simulink model "test_mdl1"  (R2023a)
settings: Solver=VariableStepAuto  StartTime=0.0  StopTime=10.0  RelTol=1e-3
(part 1 of 8)
settings Model: Creator=smqwzy  LastModifiedBy=smqwzy

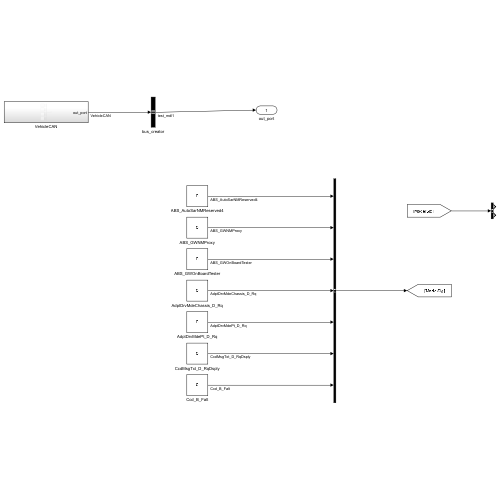
[thumbnail: Simulink's stored preview of the top-level diagram]
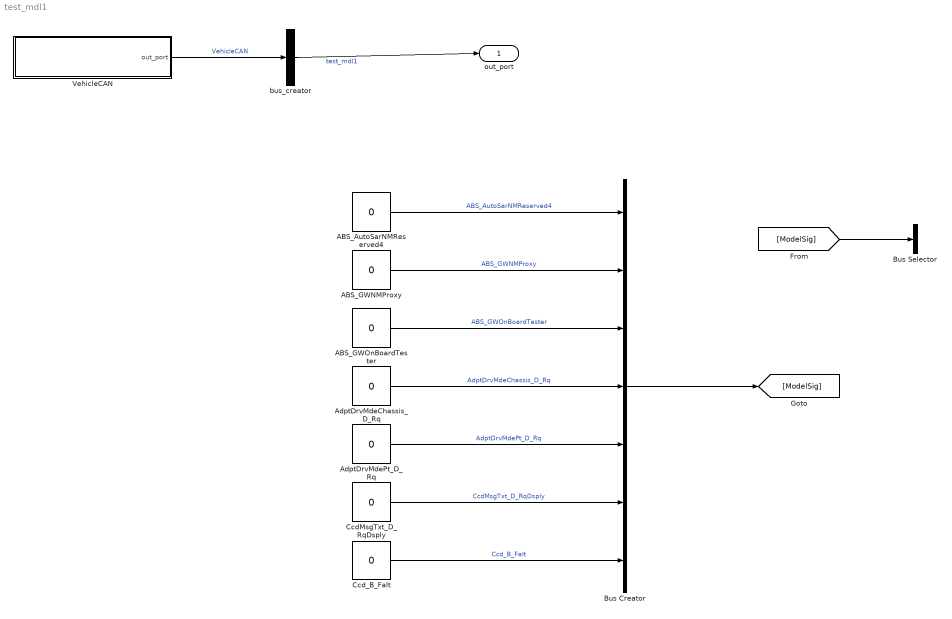
== system test_mdl1 ==
  ABS_AutoSarNMReserved4 : Constant  Value=0
  ABS_GWNMProxy : Constant  Value=0
  ABS_GWOnBoardTester : Constant  Value=0
  AdptDrvMdeChassis_D_Rq : Constant  Value=0
  AdptDrvMdePt_D_Rq : Constant  Value=0
  Bus Creator : BusCreator  Inputs=7
  Bus Selector : BusSelector  OutputSignals=signal1,signal2
  CcdMsgTxt_D_RqDsply : Constant  Value=0
  Ccd_B_Falt : Constant  Value=0
  VehicleCAN : Subsystem
  bus_creator : BusCreator  Inputs=1
  out_port : Outport
  wires:
  bus_creator/1 -> out_port/1  "test_mdl1"
  VehicleCAN/1(out_port) -> bus_creator/1  "VehicleCAN"
  Bus Creator/1 -> [ModelSig]
  [ModelSig] -> Bus Selector/1
  ABS_GWNMProxy/1 -> Bus Creator/2  "ABS_GWNMProxy"
  ABS_GWOnBoardTester/1 -> Bus Creator/3  "ABS_GWOnBoardTester"
  AdptDrvMdeChassis_D_Rq/1 -> Bus Creator/4  "AdptDrvMdeChassis_D_Rq"
  AdptDrvMdePt_D_Rq/1 -> Bus Creator/5  "AdptDrvMdePt_D_Rq"
  CcdMsgTxt_D_RqDsply/1 -> Bus Creator/6  "CcdMsgTxt_D_RqDsply"
  Ccd_B_Falt/1 -> Bus Creator/7  "Ccd_B_Falt"
  ABS_AutoSarNMReserved4/1 -> Bus Creator/1  "ABS_AutoSarNMReserved4"

== system test_mdl1/VehicleCAN ==
  ABS_ESC : Subsystem
  CMR_DSMC : Subsystem
  ECM_Diesel : Subsystem
  GWM : Subsystem
  IPMA_ADAS : Subsystem
  PCM : Subsystem
  PCM_HEV : Subsystem
  PSCM : Subsystem
  SOBDMC_HPCM_FD1 : Subsystem
  TCCM : Subsystem
  TCM_DSL : Subsystem
  TSTR : Subsystem
  VDM : Subsystem
  bus_creator : BusCreator  Inputs=13
  out_port : Outport
  wires:
  bus_creator/1 -> out_port/1  "test_mdl1"
  ABS_ESC/1(out_port) -> bus_creator/1  "ABS_ESC"
  CMR_DSMC/1(out_port) -> bus_creator/2  "CMR_DSMC"
  ECM_Diesel/1(out_port) -> bus_creator/3  "ECM_Diesel"
  GWM/1(out_port) -> bus_creator/4  "GWM"
  IPMA_ADAS/1(out_port) -> bus_creator/5  "IPMA_ADAS"
  PCM/1(out_port) -> bus_creator/6  "PCM"
  PCM_HEV/1(out_port) -> bus_creator/7  "PCM_HEV"
  PSCM/1(out_port) -> bus_creator/8  "PSCM"
  SOBDMC_HPCM_FD1/1(out_port) -> bus_creator/9  "SOBDMC_HPCM_FD1"
  TCCM/1(out_port) -> bus_creator/10  "TCCM"
  TCM_DSL/1(out_port) -> bus_creator/11  "TCM_DSL"
  TSTR/1(out_port) -> bus_creator/12  "TSTR"
  VDM/1(out_port) -> bus_creator/13  "VDM"

== system test_mdl1/VehicleCAN/ABS_ESC ==
  ABS_AutoSar_NetworkMgt : Subsystem
  ABS_BrkBst_Data : Subsystem
  ABS_Rapid_Data_Response_1 : Subsystem
  ABS_Rapid_Data_Response_2 : Subsystem
  ActiveFronSteering_Req : Subsystem
  BrakeSnData_3 : Subsystem
  BrakeSnData_4 : Subsystem
  BrakeSnData_5 : Subsystem
  BrakeSnData_6 : Subsystem
  BrakeSysFeatures : Subsystem
  BrakeSysFeatures_2 : Subsystem
  BrakeSysFeatures_3 : Subsystem
  DesiredTorqBrk : Subsystem
  DesiredTorqBrk_2 : Subsystem
  Global_PATS_SubTarget : Subsystem
  OTAPhysABStoGWM_ECG : Subsystem
  PARSEDPhysABStoGWM_ECG : Subsystem
  PARSEDPushABStoGWM_ECG : Subsystem
  SelectDriveModeData : Subsystem
  SelectDriveModeData2 : Subsystem
  TesterPhysicalResABS : Subsystem
  TrailerBrakeData : Subsystem
  WheelData : Subsystem
  WheelSpeed : Subsystem
  bus_creator : BusCreator  Inputs=24
  out_port : Outport
  wires:
  bus_creator/1 -> out_port/1  "test_mdl1"
  ABS_AutoSar_NetworkMgt/1(out_port) -> bus_creator/1  "ABS_AutoSar_NetworkMgt"
  ABS_BrkBst_Data/1(out_port) -> bus_creator/2  "ABS_BrkBst_Data"
  ABS_Rapid_Data_Response_1/1(out_port) -> bus_creator/3  "ABS_Rapid_Data_Response_1"
  ABS_Rapid_Data_Response_2/1(out_port) -> bus_creator/4  "ABS_Rapid_Data_Response_2"
  ActiveFronSteering_Req/1(out_port) -> bus_creator/5  "ActiveFronSteering_Req"
  BrakeSnData_3/1(out_port) -> bus_creator/6  "BrakeSnData_3"
  BrakeSnData_4/1(out_port) -> bus_creator/7  "BrakeSnData_4"
  BrakeSnData_5/1(out_port) -> bus_creator/8  "BrakeSnData_5"
  BrakeSnData_6/1(out_port) -> bus_creator/9  "BrakeSnData_6"
  BrakeSysFeatures/1(out_port) -> bus_creator/10  "BrakeSysFeatures"
  BrakeSysFeatures_2/1(out_port) -> bus_creator/11  "BrakeSysFeatures_2"
  BrakeSysFeatures_3/1(out_port) -> bus_creator/12  "BrakeSysFeatures_3"
  DesiredTorqBrk/1(out_port) -> bus_creator/13  "DesiredTorqBrk"
  DesiredTorqBrk_2/1(out_port) -> bus_creator/14  "DesiredTorqBrk_2"
  Global_PATS_SubTarget/1(out_port) -> bus_creator/15  "Global_PATS_SubTarget"
  OTAPhysABStoGWM_ECG/1(out_port) -> bus_creator/16  "OTAPhysABStoGWM_ECG"
  PARSEDPhysABStoGWM_ECG/1(out_port) -> bus_creator/17  "PARSEDPhysABStoGWM_ECG"
  PARSEDPushABStoGWM_ECG/1(out_port) -> bus_creator/18  "PARSEDPushABStoGWM_ECG"
  SelectDriveModeData/1(out_port) -> bus_creator/19  "SelectDriveModeData"
  SelectDriveModeData2/1(out_port) -> bus_creator/20  "SelectDriveModeData2"
  TesterPhysicalResABS/1(out_port) -> bus_creator/21  "TesterPhysicalResABS"
  TrailerBrakeData/1(out_port) -> bus_creator/22  "TrailerBrakeData"
  WheelData/1(out_port) -> bus_creator/23  "WheelData"
  WheelSpeed/1(out_port) -> bus_creator/24  "WheelSpeed"

== system test_mdl1/VehicleCAN/CMR_DSMC ==
  CMR_DSMC_AutoSar_NetwrkMgt : Subsystem
  DrvStatMonData : Subsystem
  TesterPhysicalResCMR_DSMC : Subsystem
  bus_creator : BusCreator  Inputs=3
  out_port : Outport
  wires:
  bus_creator/1 -> out_port/1  "test_mdl1"
  CMR_DSMC_AutoSar_NetwrkMgt/1(out_port) -> bus_creator/1  "CMR_DSMC_AutoSar_NetwrkMgt"
  DrvStatMonData/1(out_port) -> bus_creator/2  "DrvStatMonData"
  TesterPhysicalResCMR_DSMC/1(out_port) -> bus_creator/3  "TesterPhysicalResCMR_DSMC"

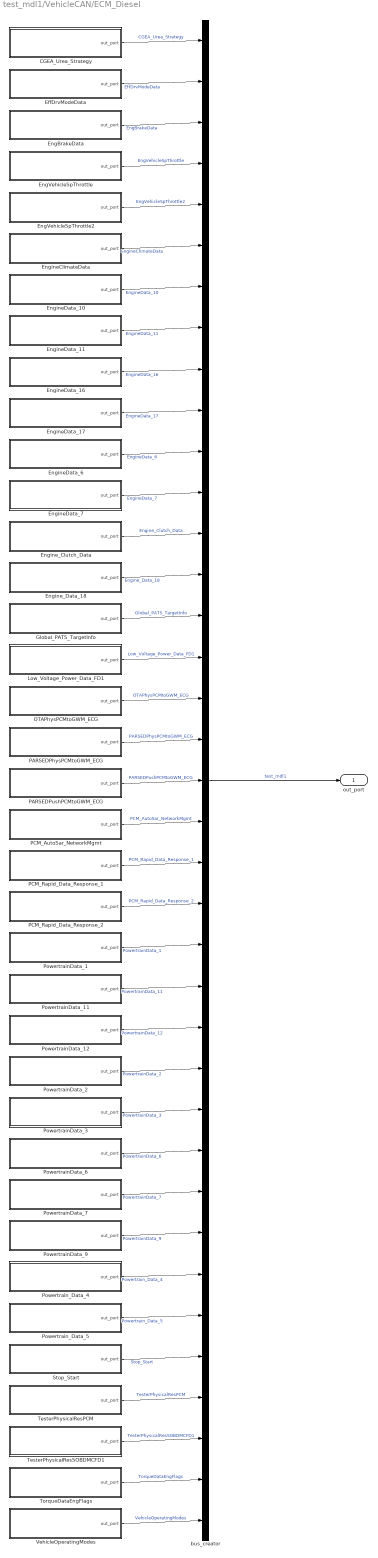
== system test_mdl1/VehicleCAN/ECM_Diesel ==
  CGEA_Urea_Strategy : Subsystem
  EffDrvModeData : Subsystem
  EngBrakeData : Subsystem
  EngVehicleSpThrottle : Subsystem
  EngVehicleSpThrottle2 : Subsystem
  EngineClimateData : Subsystem
  EngineData_10 : Subsystem
  EngineData_11 : Subsystem
  EngineData_16 : Subsystem
  EngineData_17 : Subsystem
  EngineData_6 : Subsystem
  EngineData_7 : Subsystem
  Engine_Clutch_Data : Subsystem
  Engine_Data_18 : Subsystem
  Global_PATS_TargetInfo : Subsystem
  Low_Voltage_Power_Data_FD1 : Subsystem
  OTAPhysPCMtoGWM_ECG : Subsystem
  PARSEDPhysPCMtoGWM_ECG : Subsystem
  PARSEDPushPCMtoGWM_ECG : Subsystem
  PCM_AutoSar_NetworkMgmt : Subsystem
  PCM_Rapid_Data_Response_1 : Subsystem
  PCM_Rapid_Data_Response_2 : Subsystem
  PowertrainData_1 : Subsystem
  PowertrainData_11 : Subsystem
  PowertrainData_12 : Subsystem
  PowertrainData_2 : Subsystem
  PowertrainData_3 : Subsystem
  PowertrainData_6 : Subsystem
  PowertrainData_7 : Subsystem
  PowertrainData_9 : Subsystem
  Powertrain_Data_4 : Subsystem
  Powertrain_Data_5 : Subsystem
  Stop_Start : Subsystem
  TesterPhysicalResPCM : Subsystem
  TesterPhysicalResSOBDMCFD1 : Subsystem
  TorqueDataEngFlags : Subsystem
  VehicleOperatingModes : Subsystem
  bus_creator : BusCreator  Inputs=37
  out_port : Outport
  wires:
  bus_creator/1 -> out_port/1  "test_mdl1"
  CGEA_Urea_Strategy/1(out_port) -> bus_creator/1  "CGEA_Urea_Strategy"
  EffDrvModeData/1(out_port) -> bus_creator/2  "EffDrvModeData"
  EngBrakeData/1(out_port) -> bus_creator/3  "EngBrakeData"
  EngVehicleSpThrottle/1(out_port) -> bus_creator/4  "EngVehicleSpThrottle"
  EngVehicleSpThrottle2/1(out_port) -> bus_creator/5  "EngVehicleSpThrottle2"
  EngineClimateData/1(out_port) -> bus_creator/6  "EngineClimateData"
  EngineData_10/1(out_port) -> bus_creator/7  "EngineData_10"
  EngineData_11/1(out_port) -> bus_creator/8  "EngineData_11"
  EngineData_16/1(out_port) -> bus_creator/9  "EngineData_16"
  EngineData_17/1(out_port) -> bus_creator/10  "EngineData_17"
  EngineData_6/1(out_port) -> bus_creator/11  "EngineData_6"
  EngineData_7/1(out_port) -> bus_creator/12  "EngineData_7"
  Engine_Clutch_Data/1(out_port) -> bus_creator/13  "Engine_Clutch_Data"
  Engine_Data_18/1(out_port) -> bus_creator/14  "Engine_Data_18"
  Global_PATS_TargetInfo/1(out_port) -> bus_creator/15  "Global_PATS_TargetInfo"
  Low_Voltage_Power_Data_FD1/1(out_port) -> bus_creator/16  "Low_Voltage_Power_Data_FD1"
  OTAPhysPCMtoGWM_ECG/1(out_port) -> bus_creator/17  "OTAPhysPCMtoGWM_ECG"
  PARSEDPhysPCMtoGWM_ECG/1(out_port) -> bus_creator/18  "PARSEDPhysPCMtoGWM_ECG"
  PARSEDPushPCMtoGWM_ECG/1(out_port) -> bus_creator/19  "PARSEDPushPCMtoGWM_ECG"
  PCM_AutoSar_NetworkMgmt/1(out_port) -> bus_creator/20  "PCM_AutoSar_NetworkMgmt"
  PCM_Rapid_Data_Response_1/1(out_port) -> bus_creator/21  "PCM_Rapid_Data_Response_1"
  PCM_Rapid_Data_Response_2/1(out_port) -> bus_creator/22  "PCM_Rapid_Data_Response_2"
  PowertrainData_1/1(out_port) -> bus_creator/23  "PowertrainData_1"
  PowertrainData_11/1(out_port) -> bus_creator/24  "PowertrainData_11"
  PowertrainData_12/1(out_port) -> bus_creator/25  "PowertrainData_12"
  PowertrainData_2/1(out_port) -> bus_creator/26  "PowertrainData_2"
  PowertrainData_3/1(out_port) -> bus_creator/27  "PowertrainData_3"
  PowertrainData_6/1(out_port) -> bus_creator/28  "PowertrainData_6"
  PowertrainData_7/1(out_port) -> bus_creator/29  "PowertrainData_7"
  PowertrainData_9/1(out_port) -> bus_creator/30  "PowertrainData_9"
  Powertrain_Data_4/1(out_port) -> bus_creator/31  "Powertrain_Data_4"
  Powertrain_Data_5/1(out_port) -> bus_creator/32  "Powertrain_Data_5"
  Stop_Start/1(out_port) -> bus_creator/33  "Stop_Start"
  TesterPhysicalResPCM/1(out_port) -> bus_creator/34  "TesterPhysicalResPCM"
  TesterPhysicalResSOBDMCFD1/1(out_port) -> bus_creator/35  "TesterPhysicalResSOBDMCFD1"
  TorqueDataEngFlags/1(out_port) -> bus_creator/36  "TorqueDataEngFlags"
  VehicleOperatingModes/1(out_port) -> bus_creator/37  "VehicleOperatingModes"

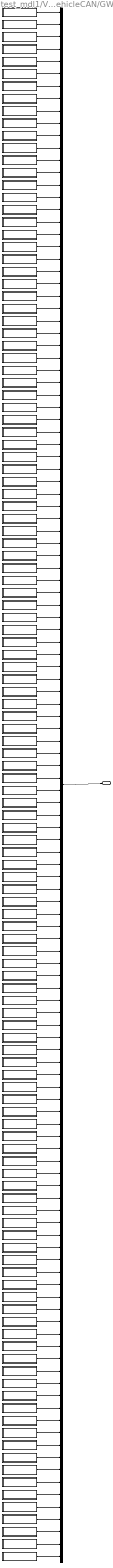
== system test_mdl1/VehicleCAN/GWM ==
  %sonality_APIM_Data_FD1 : Subsystem
  %sonality_BCM2_Data_FD1 : Subsystem
  %sonality_Data_FD1 : Subsystem
  AC_Compressor_Data_FD1 : Subsystem
  APIMGPS_Data_Nav_1_FD1 : Subsystem
  APIMGPS_Data_Nav_2_FD1 : Subsystem
  APIMGPS_Data_Nav_3_FD1 : Subsystem
  APIM_Data_FD1 : Subsystem
  APIM_Request_Signals_1_FD1 : Subsystem
  APIM_Request_Signals_5_FD1 : Subsystem
  APIM_Request_Signals_FD1 : Subsystem
  APIM_Send_Signals1_FD1 : Subsystem
  APIM_Send_Signals_2_FD1 : Subsystem
  Accel_Data_FD1 : Subsystem
  ActiveFrontStrg_Stat2_FD1 : Subsystem
  ActiveFrontStrg_Stat_FD1 : Subsystem
  Adaptive_Headlamp_Stat : Subsystem
  AllTerrainControlData_FD1 : Subsystem
  All_Terrain_Data_FD1 : Subsystem
  BCMC_Data_FD1 : Subsystem
  BCM_Lamp_Stat_FD1 : Subsystem
  BattRgenLo_1_FD1 : Subsystem
  BattRgenLo_2_FD1 : Subsystem
  BattRgenLo_3_FD1 : Subsystem
  BattRgenLo_4_FD1 : Subsystem
  Battery_Mgmt_24V_FD1 : Subsystem
  Battery_Mgmt_2_FD1 : Subsystem
  Battery_Mgmt_3_FD1 : Subsystem
  Battery_Mgmt_4_FD1 : Subsystem
  Battery_Traction_1_FD1 : Subsystem
  Battery_Traction_3_FD1 : Subsystem
  Battery_Traction_4_FD1 : Subsystem
  Battery_Traction_5_FD1 : Subsystem
  Battery_Traction_6_FD1 : Subsystem
  BodyInfo_3_FD1 : Subsystem
  Body_Info_10_FD1 : Subsystem
  Body_Info_4_FD1 : Subsystem
  Body_Info_6_FD1 : Subsystem
  Body_Info_8_FD1 : Subsystem
  Body_Info_9_FD1 : Subsystem
  Climate_Cntrl_Data_2_FD1 : Subsystem
  Climate_Control_Data_FD1 : Subsystem
  Cluster_HEV_Data8_FD1 : Subsystem
  Cluster_Info1_FD1 : Subsystem
  Cluster_Info_3_FD1 : Subsystem
  Cluster_Lighting_Rq_FD1 : Subsystem
  Compressor_Req_FD1 : Subsystem
  CruiseCtrl_Strg_Data_FD1 : Subsystem
  DCACA_Data1_FD1 : Subsystem
  DCACA_Data2_FD1 : Subsystem
  DCACA_Data3_FD1 : Subsystem
  DTE_ECGtoHPCM : Subsystem
  Driver_Dr_Stat_FD1 : Subsystem
  Dsp_Request_Signals11_FD1 : Subsystem
  ECG_Data2_FD1 : Subsystem
  ECG_Data3_FD1 : Subsystem
  ECG_Data4_FD1 : Subsystem
  ECG_Data_FD1 : Subsystem
  ElecHorizon_Data1_FD1 : Subsystem
  ElecHorizon_Data2_FD1 : Subsystem
  FourByFourSwitchData_FD1 : Subsystem
  GGCC_Config_Mgmt_ID_1_FD1 : Subsystem
  GWM_AutoSar_NetMgmt_FD1 : Subsystem
  Gear_Shift_by_Wire_2_FD1 : Subsystem
  Gear_Shift_by_Wire_FD1 : Subsystem
  GlobalClock_Data_FD1 : Subsystem
  Global_PATS_Cntrl_Info_FD1 : Subsystem
  Global_PATS_Ctrl_Info2_FD1 : Subsystem
  HeadUpDisplayReq_FD1 : Subsystem
  IPC_Infotainment_FD1 : Subsystem
  IPC_Send_Signals_2_FD1 : Subsystem
  LocationServices_3_FD1 : Subsystem
  LocationServices_Data1_FD1 : Subsystem
  Locking_Systems_2_FD1 : Subsystem
  MasterReset_HS3_ECGDat_FD1 : Subsystem
  Mc_Send_Signals_2_FD1 : Subsystem
  OTAFuncGWM_ECG_FD1 : Subsystem
  OTAPhysGWM_ECGtoABS : Subsystem
  OTAPhysGWM_ECGtoCCM : Subsystem
  OTAPhysGWM_ECGtoIPMA : Subsystem
  OTAPhysGWM_ECGtoPCM : Subsystem
  OTAPhysGWM_ECGtoSOBDMC_FD1 : Subsystem
  OTAPhysGWM_ECGtoSODCMC : Subsystem
  OTAPhysGWM_ECGtoSODCMD : Subsystem
  OTAPhysGWM_ECGtoSODL : Subsystem
  OTAPhysGWM_ECGtoSODR : Subsystem
  OffBrdChrg_Signals : Subsystem
  OffBrdChrg_Signals2 : Subsystem
  PARSEDFuncGWM_ECG_FD1 : Subsystem
  PARSEDPhysGWM_ECGtoABS : Subsystem
  PARSEDPhysGWM_ECGtoCCM : Subsystem
  PARSEDPhysGWM_ECGtoIPMA : Subsystem
  PARSEDPhysGWM_ECGtoPCM : Subsystem
  PARSEDPhysGWM_ECGtoSODCMC : Subsystem
  PARSEDPhysGWM_ECGtoSODCMD : Subsystem
  PARSEDPhysGWM_ECGtoSODL : Subsystem
  PARSEDPhysGWM_ECGtoSODR : Subsystem
  PARSEDPhysGWMtoSOBDMC_FD1 : Subsystem
  PARSEDPushFcGWM_ECGtoABS : Subsystem
  PARSEDPushFcGWM_ECGtoPCM : Subsystem
  PHEV_Battery_Data1_FD1 : Subsystem
  ParkAid_Aud_Warn_CmdM_FD1 : Subsystem
  Pass_Dr_Stat_FD1 : Subsystem
  PowerDistData_2_FD1 : Subsystem
  PowerDist_Data1_FD1 : Subsystem
  Power_Liftgate_Stat_FD1 : Subsystem
  RCMSerialNumber_FD1 : Subsystem
  RCMStatusMessage2_FD1 : Subsystem
  SmartChargingData_ECG_1 : Subsystem
  SmartChargingData_ECG_2 : Subsystem
  SmartChargingData_ECG_3 : Subsystem
  Steering_Data_FD1 : Subsystem
  Steering_Wheel_Data2_FD1 : Subsystem
  TCU_Send_Signals_FD1 : Subsystem
  TesterPhysicalReqVDM_FD1 : Subsystem
  TesterPhysicalResGWM_FD1 : Subsystem
  Tire_Pressure_Data_FD1 : Subsystem
  TrailerAid_Data3_FD1 : Subsystem
  TrailerAid_Data_FD1 : Subsystem
  TrailerAid_Stat1_FD1 : Subsystem
  TrailerAid_Stat2_FD1 : Subsystem
  TrailerBrakeInfo_FD1 : Subsystem
  TrailerInfo_2_FD1 : Subsystem
  TrailerInfo_FD1 : Subsystem
  Voltage_Power_Data2_FD1 : Subsystem
  Yaw_Data_FD1 : Subsystem
  bus_creator : BusCreator  Inputs=126
  out_port : Outport
  wires:
  bus_creator/1 -> out_port/1  "test_mdl1"
  AC_Compressor_Data_FD1/1(out_port) -> bus_creator/1  "AC_Compressor_Data_FD1"
  APIMGPS_Data_Nav_1_FD1/1(out_port) -> bus_creator/2  "APIMGPS_Data_Nav_1_FD1"
  APIMGPS_Data_Nav_2_FD1/1(out_port) -> bus_creator/3  "APIMGPS_Data_Nav_2_FD1"
  APIMGPS_Data_Nav_3_FD1/1(out_port) -> bus_creator/4  "APIMGPS_Data_Nav_3_FD1"
  APIM_Data_FD1/1(out_port) -> bus_creator/5  "APIM_Data_FD1"
  APIM_Request_Signals_1_FD1/1(out_port) -> bus_creator/6  "APIM_Request_Signals_1_FD1"
  APIM_Request_Signals_5_FD1/1(out_port) -> bus_creator/7  "APIM_Request_Signals_5_FD1"
  APIM_Request_Signals_FD1/1(out_port) -> bus_creator/8  "APIM_Request_Signals_FD1"
  APIM_Send_Signals1_FD1/1(out_port) -> bus_creator/9  "APIM_Send_Signals1_FD1"
  APIM_Send_Signals_2_FD1/1(out_port) -> bus_creator/10  "APIM_Send_Signals_2_FD1"
  Accel_Data_FD1/1(out_port) -> bus_creator/11  "Accel_Data_FD1"
  ActiveFrontStrg_Stat2_FD1/1(out_port) -> bus_creator/12  "ActiveFrontStrg_Stat2_FD1"
  ActiveFrontStrg_Stat_FD1/1(out_port) -> bus_creator/13  "ActiveFrontStrg_Stat_FD1"
  Adaptive_Headlamp_Stat/1(out_port) -> bus_creator/14  "Adaptive_Headlamp_Stat"
  AllTerrainControlData_FD1/1(out_port) -> bus_creator/15  "AllTerrainControlData_FD1"
  All_Terrain_Data_FD1/1(out_port) -> bus_creator/16  "All_Terrain_Data_FD1"
  BCMC_Data_FD1/1(out_port) -> bus_creator/17  "BCMC_Data_FD1"
  BCM_Lamp_Stat_FD1/1(out_port) -> bus_creator/18  "BCM_Lamp_Stat_FD1"
  BattRgenLo_1_FD1/1(out_port) -> bus_creator/19  "BattRgenLo_1_FD1"
  BattRgenLo_2_FD1/1(out_port) -> bus_creator/20  "BattRgenLo_2_FD1"
  BattRgenLo_3_FD1/1(out_port) -> bus_creator/21  "BattRgenLo_3_FD1"
  BattRgenLo_4_FD1/1(out_port) -> bus_creator/22  "BattRgenLo_4_FD1"
  Battery_Mgmt_24V_FD1/1(out_port) -> bus_creator/23  "Battery_Mgmt_24V_FD1"
  Battery_Mgmt_2_FD1/1(out_port) -> bus_creator/24  "Battery_Mgmt_2_FD1"
  Battery_Mgmt_3_FD1/1(out_port) -> bus_creator/25  "Battery_Mgmt_3_FD1"
  Battery_Mgmt_4_FD1/1(out_port) -> bus_creator/26  "Battery_Mgmt_4_FD1"
  Battery_Traction_1_FD1/1(out_port) -> bus_creator/27  "Battery_Traction_1_FD1"
  Battery_Traction_3_FD1/1(out_port) -> bus_creator/28  "Battery_Traction_3_FD1"
  Battery_Traction_4_FD1/1(out_port) -> bus_creator/29  "Battery_Traction_4_FD1"
  Battery_Traction_5_FD1/1(out_port) -> bus_creator/30  "Battery_Traction_5_FD1"
  Battery_Traction_6_FD1/1(out_port) -> bus_creator/31  "Battery_Traction_6_FD1"
  BodyInfo_3_FD1/1(out_port) -> bus_creator/32  "BodyInfo_3_FD1"
  Body_Info_10_FD1/1(out_port) -> bus_creator/33  "Body_Info_10_FD1"
  Body_Info_4_FD1/1(out_port) -> bus_creator/34  "Body_Info_4_FD1"
  Body_Info_6_FD1/1(out_port) -> bus_creator/35  "Body_Info_6_FD1"
  Body_Info_8_FD1/1(out_port) -> bus_creator/36  "Body_Info_8_FD1"
  Body_Info_9_FD1/1(out_port) -> bus_creator/37  "Body_Info_9_FD1"
  Climate_Cntrl_Data_2_FD1/1(out_port) -> bus_creator/38  "Climate_Cntrl_Data_2_FD1"
  Climate_Control_Data_FD1/1(out_port) -> bus_creator/39  "Climate_Control_Data_FD1"
  Cluster_HEV_Data8_FD1/1(out_port) -> bus_creator/40  "Cluster_HEV_Data8_FD1"
  Cluster_Info1_FD1/1(out_port) -> bus_creator/41  "Cluster_Info1_FD1"
  Cluster_Info_3_FD1/1(out_port) -> bus_creator/42  "Cluster_Info_3_FD1"
  Cluster_Lighting_Rq_FD1/1(out_port) -> bus_creator/43  "Cluster_Lighting_Rq_FD1"
  Compressor_Req_FD1/1(out_port) -> bus_creator/44  "Compressor_Req_FD1"
  CruiseCtrl_Strg_Data_FD1/1(out_port) -> bus_creator/45  "CruiseCtrl_Strg_Data_FD1"
  DCACA_Data1_FD1/1(out_port) -> bus_creator/46  "DCACA_Data1_FD1"
  DCACA_Data2_FD1/1(out_port) -> bus_creator/47  "DCACA_Data2_FD1"
  DCACA_Data3_FD1/1(out_port) -> bus_creator/48  "DCACA_Data3_FD1"
  DTE_ECGtoHPCM/1(out_port) -> bus_creator/49  "DTE_ECGtoHPCM"
  Driver_Dr_Stat_FD1/1(out_port) -> bus_creator/50  "Driver_Dr_Stat_FD1"
  Dsp_Request_Signals11_FD1/1(out_port) -> bus_creator/51  "Dsp_Request_Signals11_FD1"
  ECG_Data2_FD1/1(out_port) -> bus_creator/52  "ECG_Data2_FD1"
  ECG_Data3_FD1/1(out_port) -> bus_creator/53  "ECG_Data3_FD1"
  ECG_Data4_FD1/1(out_port) -> bus_creator/54  "ECG_Data4_FD1"
  ECG_Data_FD1/1(out_port) -> bus_creator/55  "ECG_Data_FD1"
  ElecHorizon_Data1_FD1/1(out_port) -> bus_creator/56  "ElecHorizon_Data1_FD1"
  ElecHorizon_Data2_FD1/1(out_port) -> bus_creator/57  "ElecHorizon_Data2_FD1"
  FourByFourSwitchData_FD1/1(out_port) -> bus_creator/58  "FourByFourSwitchData_FD1"
  GGCC_Config_Mgmt_ID_1_FD1/1(out_port) -> bus_creator/59  "GGCC_Config_Mgmt_ID_1_FD1"
  GWM_AutoSar_NetMgmt_FD1/1(out_port) -> bus_creator/60  "GWM_AutoSar_NetMgmt_FD1"
  Gear_Shift_by_Wire_2_FD1/1(out_port) -> bus_creator/61  "Gear_Shift_by_Wire_2_FD1"
  Gear_Shift_by_Wire_FD1/1(out_port) -> bus_creator/62  "Gear_Shift_by_Wire_FD1"
  GlobalClock_Data_FD1/1(out_port) -> bus_creator/63  "GlobalClock_Data_FD1"
  Global_PATS_Cntrl_Info_FD1/1(out_port) -> bus_creator/64  "Global_PATS_Cntrl_Info_FD1"
  Global_PATS_Ctrl_Info2_FD1/1(out_port) -> bus_creator/65  "Global_PATS_Ctrl_Info2_FD1"
  HeadUpDisplayReq_FD1/1(out_port) -> bus_creator/66  "HeadUpDisplayReq_FD1"
  IPC_Infotainment_FD1/1(out_port) -> bus_creator/67  "IPC_Infotainment_FD1"
  IPC_Send_Signals_2_FD1/1(out_port) -> bus_creator/68  "IPC_Send_Signals_2_FD1"
  LocationServices_3_FD1/1(out_port) -> bus_creator/69  "LocationServices_3_FD1"
  LocationServices_Data1_FD1/1(out_port) -> bus_creator/70  "LocationServices_Data1_FD1"
  Locking_Systems_2_FD1/1(out_port) -> bus_creator/71  "Locking_Systems_2_FD1"
  MasterReset_HS3_ECGDat_FD1/1(out_port) -> bus_creator/72  "MasterReset_HS3_ECGDat_FD1"
  Mc_Send_Signals_2_FD1/1(out_port) -> bus_creator/73  "Mc_Send_Signals_2_FD1"
  OTAFuncGWM_ECG_FD1/1(out_port) -> bus_creator/74  "OTAFuncGWM_ECG_FD1"
  OTAPhysGWM_ECGtoABS/1(out_port) -> bus_creator/75  "OTAPhysGWM_ECGtoABS"
  OTAPhysGWM_ECGtoCCM/1(out_port) -> bus_creator/76  "OTAPhysGWM_ECGtoCCM"
  OTAPhysGWM_ECGtoIPMA/1(out_port) -> bus_creator/77  "OTAPhysGWM_ECGtoIPMA"
  OTAPhysGWM_ECGtoPCM/1(out_port) -> bus_creator/78  "OTAPhysGWM_ECGtoPCM"
  OTAPhysGWM_ECGtoSOBDMC_FD1/1(out_port) -> bus_creator/79  "OTAPhysGWM_ECGtoSOBDMC_FD1"
  OTAPhysGWM_ECGtoSODCMC/1(out_port) -> bus_creator/80  "OTAPhysGWM_ECGtoSODCMC"
  OTAPhysGWM_ECGtoSODCMD/1(out_port) -> bus_creator/81  "OTAPhysGWM_ECGtoSODCMD"
  OTAPhysGWM_ECGtoSODL/1(out_port) -> bus_creator/82  "OTAPhysGWM_ECGtoSODL"
  OTAPhysGWM_ECGtoSODR/1(out_port) -> bus_creator/83  "OTAPhysGWM_ECGtoSODR"
  OffBrdChrg_Signals/1(out_port) -> bus_creator/84  "OffBrdChrg_Signals"
  OffBrdChrg_Signals2/1(out_port) -> bus_creator/85  "OffBrdChrg_Signals2"
  PARSEDFuncGWM_ECG_FD1/1(out_port) -> bus_creator/86  "PARSEDFuncGWM_ECG_FD1"
  PARSEDPhysGWM_ECGtoABS/1(out_port) -> bus_creator/87  "PARSEDPhysGWM_ECGtoABS"
  PARSEDPhysGWM_ECGtoCCM/1(out_port) -> bus_creator/88  "PARSEDPhysGWM_ECGtoCCM"
  PARSEDPhysGWM_ECGtoIPMA/1(out_port) -> bus_creator/89  "PARSEDPhysGWM_ECGtoIPMA"
  PARSEDPhysGWM_ECGtoPCM/1(out_port) -> bus_creator/90  "PARSEDPhysGWM_ECGtoPCM"
  PARSEDPhysGWM_ECGtoSODCMC/1(out_port) -> bus_creator/91  "PARSEDPhysGWM_ECGtoSODCMC"
  PARSEDPhysGWM_ECGtoSODCMD/1(out_port) -> bus_creator/92  "PARSEDPhysGWM_ECGtoSODCMD"
  PARSEDPhysGWM_ECGtoSODL/1(out_port) -> bus_creator/93  "PARSEDPhysGWM_ECGtoSODL"
  PARSEDPhysGWM_ECGtoSODR/1(out_port) -> bus_creator/94  "PARSEDPhysGWM_ECGtoSODR"
  PARSEDPhysGWMtoSOBDMC_FD1/1(out_port) -> bus_creator/95  "PARSEDPhysGWMtoSOBDMC_FD1"
  PARSEDPushFcGWM_ECGtoABS/1(out_port) -> bus_creator/96  "PARSEDPushFcGWM_ECGtoABS"
  PARSEDPushFcGWM_ECGtoPCM/1(out_port) -> bus_creator/97  "PARSEDPushFcGWM_ECGtoPCM"
  PHEV_Battery_Data1_FD1/1(out_port) -> bus_creator/98  "PHEV_Battery_Data1_FD1"
  ParkAid_Aud_Warn_CmdM_FD1/1(out_port) -> bus_creator/99  "ParkAid_Aud_Warn_CmdM_FD1"
  Pass_Dr_Stat_FD1/1(out_port) -> bus_creator/100  "Pass_Dr_Stat_FD1"
  %sonality_APIM_Data_FD1/1(out_port) -> bus_creator/101  "%sonality_APIM_Data_FD1"
  %sonality_BCM2_Data_FD1/1(out_port) -> bus_creator/102  "%sonality_BCM2_Data_FD1"
  %sonality_Data_FD1/1(out_port) -> bus_creator/103  "%sonality_Data_FD1"
  PowerDistData_2_FD1/1(out_port) -> bus_creator/104  "PowerDistData_2_FD1"
  PowerDist_Data1_FD1/1(out_port) -> bus_creator/105  "PowerDist_Data1_FD1"
  Power_Liftgate_Stat_FD1/1(out_port) -> bus_creator/106  "Power_Liftgate_Stat_FD1"
  RCMSerialNumber_FD1/1(out_port) -> bus_creator/107  "RCMSerialNumber_FD1"
  RCMStatusMessage2_FD1/1(out_port) -> bus_creator/108  "RCMStatusMessage2_FD1"
  SmartChargingData_ECG_1/1(out_port) -> bus_creator/109  "SmartChargingData_ECG_1"
  SmartChargingData_ECG_2/1(out_port) -> bus_creator/110  "SmartChargingData_ECG_2"
  SmartChargingData_ECG_3/1(out_port) -> bus_creator/111  "SmartChargingData_ECG_3"
  Steering_Data_FD1/1(out_port) -> bus_creator/112  "Steering_Data_FD1"
  Steering_Wheel_Data2_FD1/1(out_port) -> bus_creator/113  "Steering_Wheel_Data2_FD1"
  TCU_Send_Signals_FD1/1(out_port) -> bus_creator/114  "TCU_Send_Signals_FD1"
  TesterPhysicalReqVDM_FD1/1(out_port) -> bus_creator/115  "TesterPhysicalReqVDM_FD1"
  TesterPhysicalResGWM_FD1/1(out_port) -> bus_creator/116  "TesterPhysicalResGWM_FD1"
  Tire_Pressure_Data_FD1/1(out_port) -> bus_creator/117  "Tire_Pressure_Data_FD1"
  TrailerAid_Data3_FD1/1(out_port) -> bus_creator/118  "TrailerAid_Data3_FD1"
  TrailerAid_Data_FD1/1(out_port) -> bus_creator/119  "TrailerAid_Data_FD1"
  TrailerAid_Stat1_FD1/1(out_port) -> bus_creator/120  "TrailerAid_Stat1_FD1"
  TrailerAid_Stat2_FD1/1(out_port) -> bus_creator/121  "TrailerAid_Stat2_FD1"
  TrailerBrakeInfo_FD1/1(out_port) -> bus_creator/122  "TrailerBrakeInfo_FD1"
  TrailerInfo_2_FD1/1(out_port) -> bus_creator/123  "TrailerInfo_2_FD1"
  TrailerInfo_FD1/1(out_port) -> bus_creator/124  "TrailerInfo_FD1"
  Voltage_Power_Data2_FD1/1(out_port) -> bus_creator/125  "Voltage_Power_Data2_FD1"
  Yaw_Data_FD1/1(out_port) -> bus_creator/126  "Yaw_Data_FD1"

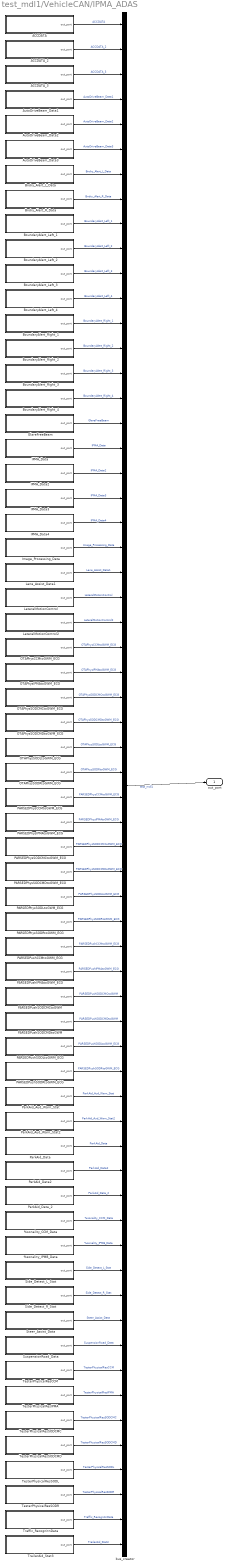
== system test_mdl1/VehicleCAN/IPMA_ADAS ==
  %sonality_CCM_Data : Subsystem
  %sonality_IPMB_Data : Subsystem
  ACCDATA : Subsystem
  ACCDATA_2 : Subsystem
  ACCDATA_3 : Subsystem
  AutoDriveBeam_Data1 : Subsystem
  AutoDriveBeam_Data2 : Subsystem
  AutoDriveBeam_Data3 : Subsystem
  Bndry_Alert_L_Data : Subsystem
  Bndry_Alert_R_Data : Subsystem
  BoundaryAlert_Left_1 : Subsystem
  BoundaryAlert_Left_2 : Subsystem
  BoundaryAlert_Left_3 : Subsystem
  BoundaryAlert_Left_4 : Subsystem
  BoundaryAlert_Right_1 : Subsystem
  BoundaryAlert_Right_2 : Subsystem
  BoundaryAlert_Right_3 : Subsystem
  BoundaryAlert_Right_4 : Subsystem
  GlareFreeBeam : Subsystem
  IPMA_Data : Subsystem
  IPMA_Data2 : Subsystem
  IPMA_Data3 : Subsystem
  IPMA_Data4 : Subsystem
  Image_Processing_Data : Subsystem
  Lane_Assist_Data1 : Subsystem
  LateralMotionControl : Subsystem
  LateralMotionControl2 : Subsystem
  OTAPhysCCMtoGWM_ECG : Subsystem
  OTAPhysIPMAtoGWM_ECG : Subsystem
  OTAPhysSODCMCtoGWM_ECG : Subsystem
  OTAPhysSODCMDtoGWM_ECG : Subsystem
  OTAPhysSODLtoGWM_ECG : Subsystem
  OTAPhysSODRtoGWM_ECG : Subsystem
  PARSEDPhysCCMtoGWM_ECG : Subsystem
  PARSEDPhysIPMAtoGWM_ECG : Subsystem
  PARSEDPhysSODCMCtoGWM_ECG : Subsystem
  PARSEDPhysSODCMDtoGWM_ECG : Subsystem
  PARSEDPhysSODLtoGWM_ECG : Subsystem
  PARSEDPhysSODRtoGWM_ECG : Subsystem
  PARSEDPushCCMtoGWM_ECG : Subsystem
  PARSEDPushIPMAtoGWM_ECG : Subsystem
  PARSEDPushSODCMCtoGWM : Subsystem
  PARSEDPushSODCMDtoGWM : Subsystem
  PARSEDPushSODLtoGWM_ECG : Subsystem
  PARSEDPushSODRtoGWM_ECG : Subsystem
  ParkAid_Aud_Warn_Stat : Subsystem
  ParkAid_Aud_Warn_Stat2 : Subsystem
  ParkAid_Data : Subsystem
  ParkAid_Data2 : Subsystem
  ParkAid_Data_2 : Subsystem
  Side_Detect_L_Stat : Subsystem
  Side_Detect_R_Stat : Subsystem
  Steer_Assist_Data : Subsystem
  SuspensionRoad_Data : Subsystem
  TesterPhysicalResCCM : Subsystem
  TesterPhysicalResIPMA : Subsystem
  TesterPhysicalResSODCMC : Subsystem
  TesterPhysicalResSODCMD : Subsystem
  TesterPhysicalResSODL : Subsystem
  TesterPhysicalResSODR : Subsystem
  Traffic_RecognitnData : Subsystem
  TrailerAid_Stat3 : Subsystem
  bus_creator : BusCreator  Inputs=62
  out_port : Outport
  wires:
  bus_creator/1 -> out_port/1  "test_mdl1"
  ACCDATA/1(out_port) -> bus_creator/1  "ACCDATA"
  ACCDATA_2/1(out_port) -> bus_creator/2  "ACCDATA_2"
  ACCDATA_3/1(out_port) -> bus_creator/3  "ACCDATA_3"
  AutoDriveBeam_Data1/1(out_port) -> bus_creator/4  "AutoDriveBeam_Data1"
  AutoDriveBeam_Data2/1(out_port) -> bus_creator/5  "AutoDriveBeam_Data2"
  AutoDriveBeam_Data3/1(out_port) -> bus_creator/6  "AutoDriveBeam_Data3"
  Bndry_Alert_L_Data/1(out_port) -> bus_creator/7  "Bndry_Alert_L_Data"
  Bndry_Alert_R_Data/1(out_port) -> bus_creator/8  "Bndry_Alert_R_Data"
  BoundaryAlert_Left_1/1(out_port) -> bus_creator/9  "BoundaryAlert_Left_1"
  BoundaryAlert_Left_2/1(out_port) -> bus_creator/10  "BoundaryAlert_Left_2"
  BoundaryAlert_Left_3/1(out_port) -> bus_creator/11  "BoundaryAlert_Left_3"
  BoundaryAlert_Left_4/1(out_port) -> bus_creator/12  "BoundaryAlert_Left_4"
  BoundaryAlert_Right_1/1(out_port) -> bus_creator/13  "BoundaryAlert_Right_1"
  BoundaryAlert_Right_2/1(out_port) -> bus_creator/14  "BoundaryAlert_Right_2"
  BoundaryAlert_Right_3/1(out_port) -> bus_creator/15  "BoundaryAlert_Right_3"
  BoundaryAlert_Right_4/1(out_port) -> bus_creator/16  "BoundaryAlert_Right_4"
  GlareFreeBeam/1(out_port) -> bus_creator/17  "GlareFreeBeam"
  IPMA_Data/1(out_port) -> bus_creator/18  "IPMA_Data"
  IPMA_Data2/1(out_port) -> bus_creator/19  "IPMA_Data2"
  IPMA_Data3/1(out_port) -> bus_creator/20  "IPMA_Data3"
  IPMA_Data4/1(out_port) -> bus_creator/21  "IPMA_Data4"
  Image_Processing_Data/1(out_port) -> bus_creator/22  "Image_Processing_Data"
  Lane_Assist_Data1/1(out_port) -> bus_creator/23  "Lane_Assist_Data1"
  LateralMotionControl/1(out_port) -> bus_creator/24  "LateralMotionControl"
  LateralMotionControl2/1(out_port) -> bus_creator/25  "LateralMotionControl2"
  OTAPhysCCMtoGWM_ECG/1(out_port) -> bus_creator/26  "OTAPhysCCMtoGWM_ECG"
  OTAPhysIPMAtoGWM_ECG/1(out_port) -> bus_creator/27  "OTAPhysIPMAtoGWM_ECG"
  OTAPhysSODCMCtoGWM_ECG/1(out_port) -> bus_creator/28  "OTAPhysSODCMCtoGWM_ECG"
  OTAPhysSODCMDtoGWM_ECG/1(out_port) -> bus_creator/29  "OTAPhysSODCMDtoGWM_ECG"
  OTAPhysSODLtoGWM_ECG/1(out_port) -> bus_creator/30  "OTAPhysSODLtoGWM_ECG"
  OTAPhysSODRtoGWM_ECG/1(out_port) -> bus_creator/31  "OTAPhysSODRtoGWM_ECG"
  PARSEDPhysCCMtoGWM_ECG/1(out_port) -> bus_creator/32  "PARSEDPhysCCMtoGWM_ECG"
  PARSEDPhysIPMAtoGWM_ECG/1(out_port) -> bus_creator/33  "PARSEDPhysIPMAtoGWM_ECG"
  PARSEDPhysSODCMCtoGWM_ECG/1(out_port) -> bus_creator/34  "PARSEDPhysSODCMCtoGWM_ECG"
  PARSEDPhysSODCMDtoGWM_ECG/1(out_port) -> bus_creator/35  "PARSEDPhysSODCMDtoGWM_ECG"
  PARSEDPhysSODLtoGWM_ECG/1(out_port) -> bus_creator/36  "PARSEDPhysSODLtoGWM_ECG"
  PARSEDPhysSODRtoGWM_ECG/1(out_port) -> bus_creator/37  "PARSEDPhysSODRtoGWM_ECG"
  PARSEDPushCCMtoGWM_ECG/1(out_port) -> bus_creator/38  "PARSEDPushCCMtoGWM_ECG"
  PARSEDPushIPMAtoGWM_ECG/1(out_port) -> bus_creator/39  "PARSEDPushIPMAtoGWM_ECG"
  PARSEDPushSODCMCtoGWM/1(out_port) -> bus_creator/40  "PARSEDPushSODCMCtoGWM"
  PARSEDPushSODCMDtoGWM/1(out_port) -> bus_creator/41  "PARSEDPushSODCMDtoGWM"
  PARSEDPushSODLtoGWM_ECG/1(out_port) -> bus_creator/42  "PARSEDPushSODLtoGWM_ECG"
  PARSEDPushSODRtoGWM_ECG/1(out_port) -> bus_creator/43  "PARSEDPushSODRtoGWM_ECG"
  ParkAid_Aud_Warn_Stat/1(out_port) -> bus_creator/44  "ParkAid_Aud_Warn_Stat"
  ParkAid_Aud_Warn_Stat2/1(out_port) -> bus_creator/45  "ParkAid_Aud_Warn_Stat2"
  ParkAid_Data/1(out_port) -> bus_creator/46  "ParkAid_Data"
  ParkAid_Data2/1(out_port) -> bus_creator/47  "ParkAid_Data2"
  ParkAid_Data_2/1(out_port) -> bus_creator/48  "ParkAid_Data_2"
  %sonality_CCM_Data/1(out_port) -> bus_creator/49  "%sonality_CCM_Data"
  %sonality_IPMB_Data/1(out_port) -> bus_creator/50  "%sonality_IPMB_Data"
  Side_Detect_L_Stat/1(out_port) -> bus_creator/51  "Side_Detect_L_Stat"
  Side_Detect_R_Stat/1(out_port) -> bus_creator/52  "Side_Detect_R_Stat"
  Steer_Assist_Data/1(out_port) -> bus_creator/53  "Steer_Assist_Data"
  SuspensionRoad_Data/1(out_port) -> bus_creator/54  "SuspensionRoad_Data"
  TesterPhysicalResCCM/1(out_port) -> bus_creator/55  "TesterPhysicalResCCM"
  TesterPhysicalResIPMA/1(out_port) -> bus_creator/56  "TesterPhysicalResIPMA"
  TesterPhysicalResSODCMC/1(out_port) -> bus_creator/57  "TesterPhysicalResSODCMC"
  TesterPhysicalResSODCMD/1(out_port) -> bus_creator/58  "TesterPhysicalResSODCMD"
  TesterPhysicalResSODL/1(out_port) -> bus_creator/59  "TesterPhysicalResSODL"
  TesterPhysicalResSODR/1(out_port) -> bus_creator/60  "TesterPhysicalResSODR"
  Traffic_RecognitnData/1(out_port) -> bus_creator/61  "Traffic_RecognitnData"
  TrailerAid_Stat3/1(out_port) -> bus_creator/62  "TrailerAid_Stat3"

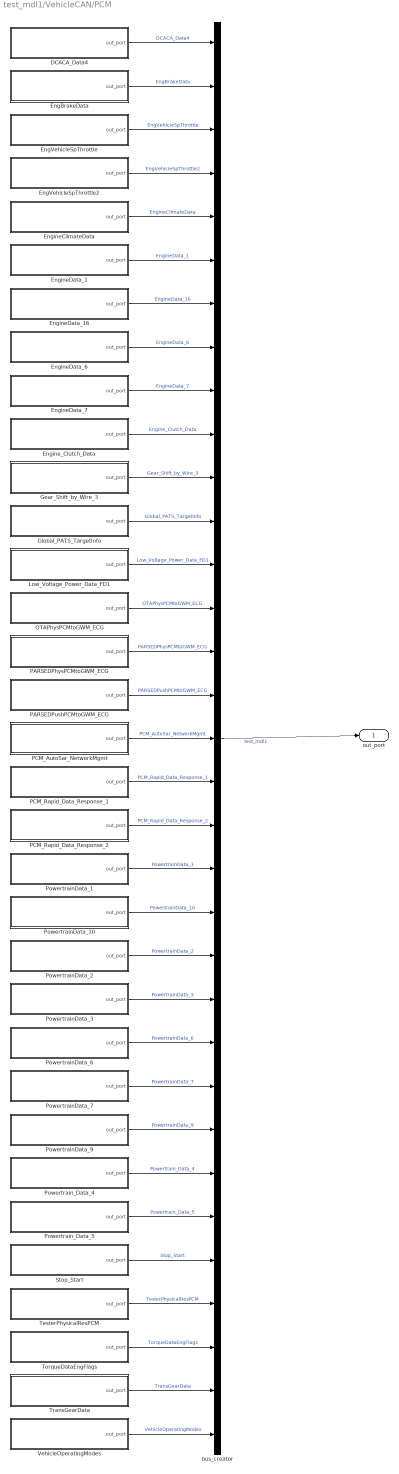
== system test_mdl1/VehicleCAN/PCM ==
  DCACA_Data4 : Subsystem
  EngBrakeData : Subsystem
  EngVehicleSpThrottle : Subsystem
  EngVehicleSpThrottle2 : Subsystem
  EngineClimateData : Subsystem
  EngineData_1 : Subsystem
  EngineData_16 : Subsystem
  EngineData_6 : Subsystem
  EngineData_7 : Subsystem
  Engine_Clutch_Data : Subsystem
  Gear_Shift_by_Wire_3 : Subsystem
  Global_PATS_TargetInfo : Subsystem
  Low_Voltage_Power_Data_FD1 : Subsystem
  OTAPhysPCMtoGWM_ECG : Subsystem
  PARSEDPhysPCMtoGWM_ECG : Subsystem
  PARSEDPushPCMtoGWM_ECG : Subsystem
  PCM_AutoSar_NetworkMgmt : Subsystem
  PCM_Rapid_Data_Response_1 : Subsystem
  PCM_Rapid_Data_Response_2 : Subsystem
  PowertrainData_1 : Subsystem
  PowertrainData_10 : Subsystem
  PowertrainData_2 : Subsystem
  PowertrainData_3 : Subsystem
  PowertrainData_6 : Subsystem
  PowertrainData_7 : Subsystem
  PowertrainData_9 : Subsystem
  Powertrain_Data_4 : Subsystem
  Powertrain_Data_5 : Subsystem
  Stop_Start : Subsystem
  TesterPhysicalResPCM : Subsystem
  TorqueDataEngFlags : Subsystem
  TransGearData : Subsystem
  VehicleOperatingModes : Subsystem
  bus_creator : BusCreator  Inputs=33
  out_port : Outport
  wires:
  bus_creator/1 -> out_port/1  "test_mdl1"
  DCACA_Data4/1(out_port) -> bus_creator/1  "DCACA_Data4"
  EngBrakeData/1(out_port) -> bus_creator/2  "EngBrakeData"
  EngVehicleSpThrottle/1(out_port) -> bus_creator/3  "EngVehicleSpThrottle"
  EngVehicleSpThrottle2/1(out_port) -> bus_creator/4  "EngVehicleSpThrottle2"
  EngineClimateData/1(out_port) -> bus_creator/5  "EngineClimateData"
  EngineData_1/1(out_port) -> bus_creator/6  "EngineData_1"
  EngineData_16/1(out_port) -> bus_creator/7  "EngineData_16"
  EngineData_6/1(out_port) -> bus_creator/8  "EngineData_6"
  EngineData_7/1(out_port) -> bus_creator/9  "EngineData_7"
  Engine_Clutch_Data/1(out_port) -> bus_creator/10  "Engine_Clutch_Data"
  Gear_Shift_by_Wire_3/1(out_port) -> bus_creator/11  "Gear_Shift_by_Wire_3"
  Global_PATS_TargetInfo/1(out_port) -> bus_creator/12  "Global_PATS_TargetInfo"
  Low_Voltage_Power_Data_FD1/1(out_port) -> bus_creator/13  "Low_Voltage_Power_Data_FD1"
  OTAPhysPCMtoGWM_ECG/1(out_port) -> bus_creator/14  "OTAPhysPCMtoGWM_ECG"
  PARSEDPhysPCMtoGWM_ECG/1(out_port) -> bus_creator/15  "PARSEDPhysPCMtoGWM_ECG"
  PARSEDPushPCMtoGWM_ECG/1(out_port) -> bus_creator/16  "PARSEDPushPCMtoGWM_ECG"
  PCM_AutoSar_NetworkMgmt/1(out_port) -> bus_creator/17  "PCM_AutoSar_NetworkMgmt"
  PCM_Rapid_Data_Response_1/1(out_port) -> bus_creator/18  "PCM_Rapid_Data_Response_1"
  PCM_Rapid_Data_Response_2/1(out_port) -> bus_creator/19  "PCM_Rapid_Data_Response_2"
  PowertrainData_1/1(out_port) -> bus_creator/20  "PowertrainData_1"
  PowertrainData_10/1(out_port) -> bus_creator/21  "PowertrainData_10"
  PowertrainData_2/1(out_port) -> bus_creator/22  "PowertrainData_2"
  PowertrainData_3/1(out_port) -> bus_creator/23  "PowertrainData_3"
  PowertrainData_6/1(out_port) -> bus_creator/24  "PowertrainData_6"
  PowertrainData_7/1(out_port) -> bus_creator/25  "PowertrainData_7"
  PowertrainData_9/1(out_port) -> bus_creator/26  "PowertrainData_9"
  Powertrain_Data_4/1(out_port) -> bus_creator/27  "Powertrain_Data_4"
  Powertrain_Data_5/1(out_port) -> bus_creator/28  "Powertrain_Data_5"
  Stop_Start/1(out_port) -> bus_creator/29  "Stop_Start"
  TesterPhysicalResPCM/1(out_port) -> bus_creator/30  "TesterPhysicalResPCM"
  TorqueDataEngFlags/1(out_port) -> bus_creator/31  "TorqueDataEngFlags"
  TransGearData/1(out_port) -> bus_creator/32  "TransGearData"
  VehicleOperatingModes/1(out_port) -> bus_creator/33  "VehicleOperatingModes"

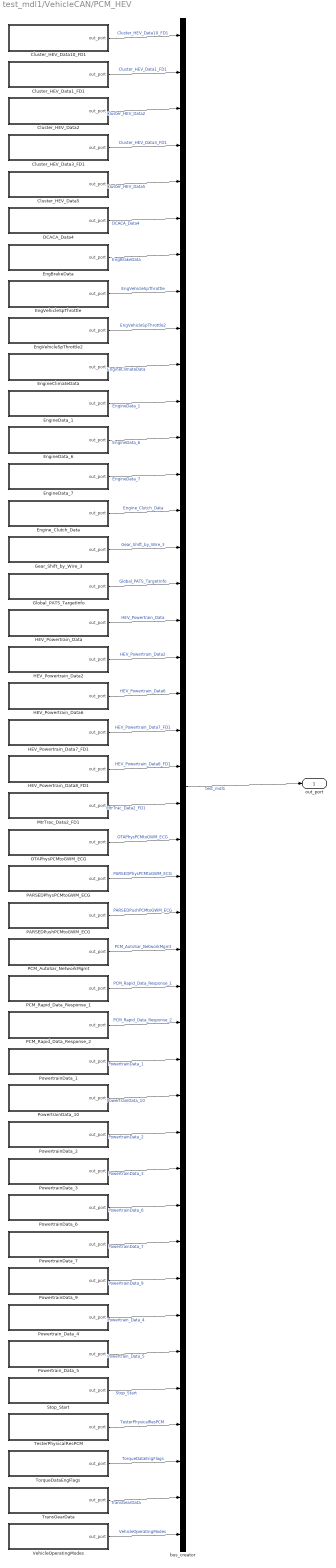
== system test_mdl1/VehicleCAN/PCM_HEV ==
  Cluster_HEV_Data10_FD1 : Subsystem
  Cluster_HEV_Data1_FD1 : Subsystem
  Cluster_HEV_Data2 : Subsystem
  Cluster_HEV_Data3_FD1 : Subsystem
  Cluster_HEV_Data5 : Subsystem
  DCACA_Data4 : Subsystem
  EngBrakeData : Subsystem
  EngVehicleSpThrottle : Subsystem
  EngVehicleSpThrottle2 : Subsystem
  EngineClimateData : Subsystem
  EngineData_1 : Subsystem
  EngineData_6 : Subsystem
  EngineData_7 : Subsystem
  Engine_Clutch_Data : Subsystem
  Gear_Shift_by_Wire_3 : Subsystem
  Global_PATS_TargetInfo : Subsystem
  HEV_Powertrain_Data : Subsystem
  HEV_Powertrain_Data2 : Subsystem
  HEV_Powertrain_Data6 : Subsystem
  HEV_Powertrain_Data7_FD1 : Subsystem
  HEV_Powertrain_Data8_FD1 : Subsystem
  MtrTrac_Data2_FD1 : Subsystem
  OTAPhysPCMtoGWM_ECG : Subsystem
  PARSEDPhysPCMtoGWM_ECG : Subsystem
  PARSEDPushPCMtoGWM_ECG : Subsystem
  PCM_AutoSar_NetworkMgmt : Subsystem
  PCM_Rapid_Data_Response_1 : Subsystem
  PCM_Rapid_Data_Response_2 : Subsystem
  PowertrainData_1 : Subsystem
  PowertrainData_10 : Subsystem
  PowertrainData_2 : Subsystem
  PowertrainData_3 : Subsystem
  PowertrainData_6 : Subsystem
  PowertrainData_7 : Subsystem
  PowertrainData_9 : Subsystem
  Powertrain_Data_4 : Subsystem
  Powertrain_Data_5 : Subsystem
  Stop_Start : Subsystem
  TesterPhysicalResPCM : Subsystem
  TorqueDataEngFlags : Subsystem
  TransGearData : Subsystem
  VehicleOperatingModes : Subsystem
  bus_creator : BusCreator  Inputs=42
  out_port : Outport
  wires:
  bus_creator/1 -> out_port/1  "test_mdl1"
  Cluster_HEV_Data10_FD1/1(out_port) -> bus_creator/1  "Cluster_HEV_Data10_FD1"
  Cluster_HEV_Data1_FD1/1(out_port) -> bus_creator/2  "Cluster_HEV_Data1_FD1"
  Cluster_HEV_Data2/1(out_port) -> bus_creator/3  "Cluster_HEV_Data2"
  Cluster_HEV_Data3_FD1/1(out_port) -> bus_creator/4  "Cluster_HEV_Data3_FD1"
  Cluster_HEV_Data5/1(out_port) -> bus_creator/5  "Cluster_HEV_Data5"
  DCACA_Data4/1(out_port) -> bus_creator/6  "DCACA_Data4"
  EngBrakeData/1(out_port) -> bus_creator/7  "EngBrakeData"
  EngVehicleSpThrottle/1(out_port) -> bus_creator/8  "EngVehicleSpThrottle"
  EngVehicleSpThrottle2/1(out_port) -> bus_creator/9  "EngVehicleSpThrottle2"
  EngineClimateData/1(out_port) -> bus_creator/10  "EngineClimateData"
  EngineData_1/1(out_port) -> bus_creator/11  "EngineData_1"
  EngineData_6/1(out_port) -> bus_creator/12  "EngineData_6"
  EngineData_7/1(out_port) -> bus_creator/13  "EngineData_7"
  Engine_Clutch_Data/1(out_port) -> bus_creator/14  "Engine_Clutch_Data"
  Gear_Shift_by_Wire_3/1(out_port) -> bus_creator/15  "Gear_Shift_by_Wire_3"
  Global_PATS_TargetInfo/1(out_port) -> bus_creator/16  "Global_PATS_TargetInfo"
  HEV_Powertrain_Data/1(out_port) -> bus_creator/17  "HEV_Powertrain_Data"
  HEV_Powertrain_Data2/1(out_port) -> bus_creator/18  "HEV_Powertrain_Data2"
  HEV_Powertrain_Data6/1(out_port) -> bus_creator/19  "HEV_Powertrain_Data6"
  HEV_Powertrain_Data7_FD1/1(out_port) -> bus_creator/20  "HEV_Powertrain_Data7_FD1"
  HEV_Powertrain_Data8_FD1/1(out_port) -> bus_creator/21  "HEV_Powertrain_Data8_FD1"
  MtrTrac_Data2_FD1/1(out_port) -> bus_creator/22  "MtrTrac_Data2_FD1"
  OTAPhysPCMtoGWM_ECG/1(out_port) -> bus_creator/23  "OTAPhysPCMtoGWM_ECG"
  PARSEDPhysPCMtoGWM_ECG/1(out_port) -> bus_creator/24  "PARSEDPhysPCMtoGWM_ECG"
  PARSEDPushPCMtoGWM_ECG/1(out_port) -> bus_creator/25  "PARSEDPushPCMtoGWM_ECG"
  PCM_AutoSar_NetworkMgmt/1(out_port) -> bus_creator/26  "PCM_AutoSar_NetworkMgmt"
  PCM_Rapid_Data_Response_1/1(out_port) -> bus_creator/27  "PCM_Rapid_Data_Response_1"
  PCM_Rapid_Data_Response_2/1(out_port) -> bus_creator/28  "PCM_Rapid_Data_Response_2"
  PowertrainData_1/1(out_port) -> bus_creator/29  "PowertrainData_1"
  PowertrainData_10/1(out_port) -> bus_creator/30  "PowertrainData_10"
  PowertrainData_2/1(out_port) -> bus_creator/31  "PowertrainData_2"
  PowertrainData_3/1(out_port) -> bus_creator/32  "PowertrainData_3"
  PowertrainData_6/1(out_port) -> bus_creator/33  "PowertrainData_6"
  PowertrainData_7/1(out_port) -> bus_creator/34  "PowertrainData_7"
  PowertrainData_9/1(out_port) -> bus_creator/35  "PowertrainData_9"
  Powertrain_Data_4/1(out_port) -> bus_creator/36  "Powertrain_Data_4"
  Powertrain_Data_5/1(out_port) -> bus_creator/37  "Powertrain_Data_5"
  Stop_Start/1(out_port) -> bus_creator/38  "Stop_Start"
  TesterPhysicalResPCM/1(out_port) -> bus_creator/39  "TesterPhysicalResPCM"
  TorqueDataEngFlags/1(out_port) -> bus_creator/40  "TorqueDataEngFlags"
  TransGearData/1(out_port) -> bus_creator/41  "TransGearData"
  VehicleOperatingModes/1(out_port) -> bus_creator/42  "VehicleOperatingModes"

== system test_mdl1/VehicleCAN/PSCM ==
  EPAS_INFO : Subsystem
  Lane_Assist_Data3_FD1 : Subsystem
  PSCM_AutoSar_NetwrkMgmt : Subsystem
  SteeringPinion_Data : Subsystem
  TesterPhysicalResPSCM : Subsystem
  TrailerAid_Data2 : Subsystem
  bus_creator : BusCreator  Inputs=6
  out_port : Outport
  wires:
  bus_creator/1 -> out_port/1  "test_mdl1"
  EPAS_INFO/1(out_port) -> bus_creator/1  "EPAS_INFO"
  Lane_Assist_Data3_FD1/1(out_port) -> bus_creator/2  "Lane_Assist_Data3_FD1"
  PSCM_AutoSar_NetwrkMgmt/1(out_port) -> bus_creator/3  "PSCM_AutoSar_NetwrkMgmt"
  SteeringPinion_Data/1(out_port) -> bus_creator/4  "SteeringPinion_Data"
  TesterPhysicalResPSCM/1(out_port) -> bus_creator/5  "TesterPhysicalResPSCM"
  TrailerAid_Data2/1(out_port) -> bus_creator/6  "TrailerAid_Data2"

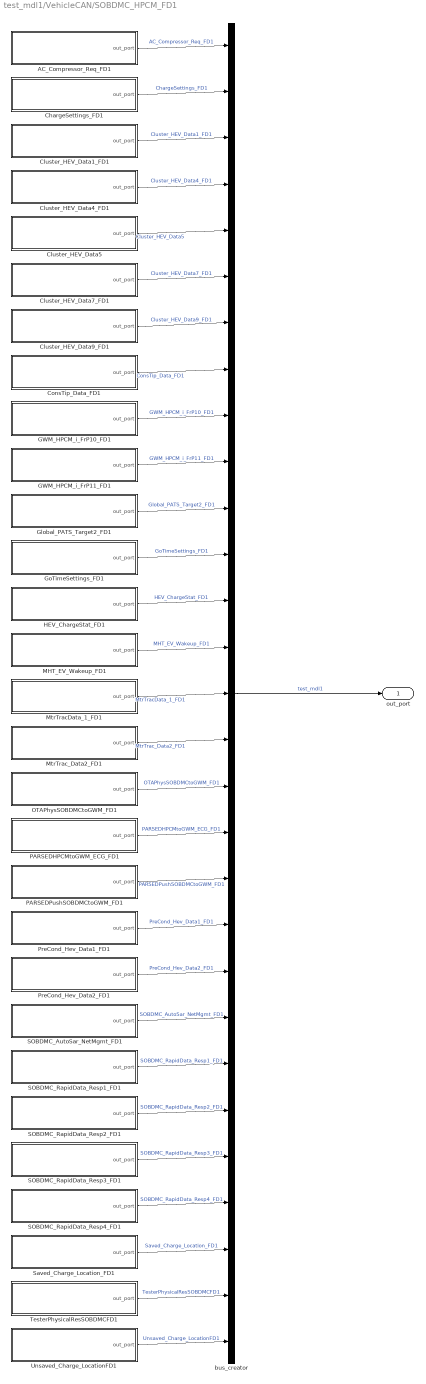
== system test_mdl1/VehicleCAN/SOBDMC_HPCM_FD1 ==
  AC_Compressor_Req_FD1 : Subsystem
  ChargeSettings_FD1 : Subsystem
  Cluster_HEV_Data1_FD1 : Subsystem
  Cluster_HEV_Data4_FD1 : Subsystem
  Cluster_HEV_Data5 : Subsystem
  Cluster_HEV_Data7_FD1 : Subsystem
  Cluster_HEV_Data9_FD1 : Subsystem
  ConsTip_Data_FD1 : Subsystem
  GWM_HPCM_i_FrP10_FD1 : Subsystem
  GWM_HPCM_i_FrP11_FD1 : Subsystem
  Global_PATS_Target2_FD1 : Subsystem
  GoTimeSettings_FD1 : Subsystem
  HEV_ChargeStat_FD1 : Subsystem
  MHT_EV_Wakeup_FD1 : Subsystem
  MtrTracData_1_FD1 : Subsystem
  MtrTrac_Data2_FD1 : Subsystem
  OTAPhysSOBDMCtoGWM_FD1 : Subsystem
  PARSEDHPCMtoGWM_ECG_FD1 : Subsystem
  PARSEDPushSOBDMCtoGWM_FD1 : Subsystem
  PreCond_Hev_Data1_FD1 : Subsystem
  PreCond_Hev_Data2_FD1 : Subsystem
  SOBDMC_AutoSar_NetMgmt_FD1 : Subsystem
  SOBDMC_RapidData_Resp1_FD1 : Subsystem
  SOBDMC_RapidData_Resp2_FD1 : Subsystem
  SOBDMC_RapidData_Resp3_FD1 : Subsystem
  SOBDMC_RapidData_Resp4_FD1 : Subsystem
  Saved_Charge_Location_FD1 : Subsystem
  TesterPhysicalResSOBDMCFD1 : Subsystem
  Unsaved_Charge_LocationFD1 : Subsystem
  bus_creator : BusCreator  Inputs=29
  out_port : Outport
  wires:
  bus_creator/1 -> out_port/1  "test_mdl1"
  AC_Compressor_Req_FD1/1(out_port) -> bus_creator/1  "AC_Compressor_Req_FD1"
  ChargeSettings_FD1/1(out_port) -> bus_creator/2  "ChargeSettings_FD1"
  Cluster_HEV_Data1_FD1/1(out_port) -> bus_creator/3  "Cluster_HEV_Data1_FD1"
  Cluster_HEV_Data4_FD1/1(out_port) -> bus_creator/4  "Cluster_HEV_Data4_FD1"
  Cluster_HEV_Data5/1(out_port) -> bus_creator/5  "Cluster_HEV_Data5"
  Cluster_HEV_Data7_FD1/1(out_port) -> bus_creator/6  "Cluster_HEV_Data7_FD1"
  Cluster_HEV_Data9_FD1/1(out_port) -> bus_creator/7  "Cluster_HEV_Data9_FD1"
  ConsTip_Data_FD1/1(out_port) -> bus_creator/8  "ConsTip_Data_FD1"
  GWM_HPCM_i_FrP10_FD1/1(out_port) -> bus_creator/9  "GWM_HPCM_i_FrP10_FD1"
  GWM_HPCM_i_FrP11_FD1/1(out_port) -> bus_creator/10  "GWM_HPCM_i_FrP11_FD1"
  Global_PATS_Target2_FD1/1(out_port) -> bus_creator/11  "Global_PATS_Target2_FD1"
  GoTimeSettings_FD1/1(out_port) -> bus_creator/12  "GoTimeSettings_FD1"
  HEV_ChargeStat_FD1/1(out_port) -> bus_creator/13  "HEV_ChargeStat_FD1"
  MHT_EV_Wakeup_FD1/1(out_port) -> bus_creator/14  "MHT_EV_Wakeup_FD1"
  MtrTracData_1_FD1/1(out_port) -> bus_creator/15  "MtrTracData_1_FD1"
  MtrTrac_Data2_FD1/1(out_port) -> bus_creator/16  "MtrTrac_Data2_FD1"
  OTAPhysSOBDMCtoGWM_FD1/1(out_port) -> bus_creator/17  "OTAPhysSOBDMCtoGWM_FD1"
  PARSEDHPCMtoGWM_ECG_FD1/1(out_port) -> bus_creator/18  "PARSEDHPCMtoGWM_ECG_FD1"
  PARSEDPushSOBDMCtoGWM_FD1/1(out_port) -> bus_creator/19  "PARSEDPushSOBDMCtoGWM_FD1"
  PreCond_Hev_Data1_FD1/1(out_port) -> bus_creator/20  "PreCond_Hev_Data1_FD1"
  PreCond_Hev_Data2_FD1/1(out_port) -> bus_creator/21  "PreCond_Hev_Data2_FD1"
  SOBDMC_AutoSar_NetMgmt_FD1/1(out_port) -> bus_creator/22  "SOBDMC_AutoSar_NetMgmt_FD1"
  SOBDMC_RapidData_Resp1_FD1/1(out_port) -> bus_creator/23  "SOBDMC_RapidData_Resp1_FD1"
  SOBDMC_RapidData_Resp2_FD1/1(out_port) -> bus_creator/24  "SOBDMC_RapidData_Resp2_FD1"
  SOBDMC_RapidData_Resp3_FD1/1(out_port) -> bus_creator/25  "SOBDMC_RapidData_Resp3_FD1"
  SOBDMC_RapidData_Resp4_FD1/1(out_port) -> bus_creator/26  "SOBDMC_RapidData_Resp4_FD1"
  Saved_Charge_Location_FD1/1(out_port) -> bus_creator/27  "Saved_Charge_Location_FD1"
  TesterPhysicalResSOBDMCFD1/1(out_port) -> bus_creator/28  "TesterPhysicalResSOBDMCFD1"
  Unsaved_Charge_LocationFD1/1(out_port) -> bus_creator/29  "Unsaved_Charge_LocationFD1"

== system test_mdl1/VehicleCAN/TCCM ==
  AWD_Torque_Data : Subsystem
  Driveline_Data_1 : Subsystem
  Driveline_Data_2 : Subsystem
  TCCM_AutoSar_NetwkMgmt : Subsystem
  TesterPhysicalResTCCM : Subsystem
  bus_creator : BusCreator  Inputs=5
  out_port : Outport
  wires:
  bus_creator/1 -> out_port/1  "test_mdl1"
  AWD_Torque_Data/1(out_port) -> bus_creator/1  "AWD_Torque_Data"
  Driveline_Data_1/1(out_port) -> bus_creator/2  "Driveline_Data_1"
  Driveline_Data_2/1(out_port) -> bus_creator/3  "Driveline_Data_2"
  TCCM_AutoSar_NetwkMgmt/1(out_port) -> bus_creator/4  "TCCM_AutoSar_NetwkMgmt"
  TesterPhysicalResTCCM/1(out_port) -> bus_creator/5  "TesterPhysicalResTCCM"

== system test_mdl1/VehicleCAN/TCM_DSL ==
  EngineData_1 : Subsystem
  Gear_Shift_by_Wire_3 : Subsystem
  PowertrainData_10 : Subsystem
  TCM_AutoSar_NetworkMgt : Subsystem
  TCM_Rapid_Data_Response_1 : Subsystem
  TCM_Rapid_Data_Response_2 : Subsystem
  TesterPhysicalResTCM : Subsystem
  TransData_3 : Subsystem
  TransGearData : Subsystem
  TransGearData_2 : Subsystem
  bus_creator : BusCreator  Inputs=10
  out_port : Outport
  wires:
  bus_creator/1 -> out_port/1  "test_mdl1"
  EngineData_1/1(out_port) -> bus_creator/1  "EngineData_1"
  Gear_Shift_by_Wire_3/1(out_port) -> bus_creator/2  "Gear_Shift_by_Wire_3"
  PowertrainData_10/1(out_port) -> bus_creator/3  "PowertrainData_10"
  TCM_AutoSar_NetworkMgt/1(out_port) -> bus_creator/4  "TCM_AutoSar_NetworkMgt"
  TCM_Rapid_Data_Response_1/1(out_port) -> bus_creator/5  "TCM_Rapid_Data_Response_1"
  TCM_Rapid_Data_Response_2/1(out_port) -> bus_creator/6  "TCM_Rapid_Data_Response_2"
  TesterPhysicalResTCM/1(out_port) -> bus_creator/7  "TesterPhysicalResTCM"
  TransData_3/1(out_port) -> bus_creator/8  "TransData_3"
  TransGearData/1(out_port) -> bus_creator/9  "TransGearData"
  TransGearData_2/1(out_port) -> bus_creator/10  "TransGearData_2"

== system test_mdl1/VehicleCAN/TSTR ==
  TesterFunctionalReq_FD1 : Subsystem
  TesterPhysicalReqABS : Subsystem
  TesterPhysicalReqCCM : Subsystem
  TesterPhysicalReqCMR_DSMC : Subsystem
  TesterPhysicalReqGWM_FD1 : Subsystem
  TesterPhysicalReqIPMA : Subsystem
  TesterPhysicalReqPCM : Subsystem
  TesterPhysicalReqPSCM : Subsystem
  TesterPhysicalReqSOBDMC_FD : Subsystem
  TesterPhysicalReqSODCMC : Subsystem
  TesterPhysicalReqSODCMD : Subsystem
  TesterPhysicalReqSODL : Subsystem
  TesterPhysicalReqSODR : Subsystem
  TesterPhysicalReqTCCM : Subsystem
  TesterPhysicalReqTCM : Subsystem
  bus_creator : BusCreator  Inputs=15
  out_port : Outport
  wires:
  bus_creator/1 -> out_port/1  "test_mdl1"
  TesterFunctionalReq_FD1/1(out_port) -> bus_creator/1  "TesterFunctionalReq_FD1"
  TesterPhysicalReqABS/1(out_port) -> bus_creator/2  "TesterPhysicalReqABS"
  TesterPhysicalReqCCM/1(out_port) -> bus_creator/3  "TesterPhysicalReqCCM"
  TesterPhysicalReqCMR_DSMC/1(out_port) -> bus_creator/4  "TesterPhysicalReqCMR_DSMC"
  TesterPhysicalReqGWM_FD1/1(out_port) -> bus_creator/5  "TesterPhysicalReqGWM_FD1"
  TesterPhysicalReqIPMA/1(out_port) -> bus_creator/6  "TesterPhysicalReqIPMA"
  TesterPhysicalReqPCM/1(out_port) -> bus_creator/7  "TesterPhysicalReqPCM"
  TesterPhysicalReqPSCM/1(out_port) -> bus_creator/8  "TesterPhysicalReqPSCM"
  TesterPhysicalReqSOBDMC_FD/1(out_port) -> bus_creator/9  "TesterPhysicalReqSOBDMC_FD"
  TesterPhysicalReqSODCMC/1(out_port) -> bus_creator/10  "TesterPhysicalReqSODCMC"
  TesterPhysicalReqSODCMD/1(out_port) -> bus_creator/11  "TesterPhysicalReqSODCMD"
  TesterPhysicalReqSODL/1(out_port) -> bus_creator/12  "TesterPhysicalReqSODL"
  TesterPhysicalReqSODR/1(out_port) -> bus_creator/13  "TesterPhysicalReqSODR"
  TesterPhysicalReqTCCM/1(out_port) -> bus_creator/14  "TesterPhysicalReqTCCM"
  TesterPhysicalReqTCM/1(out_port) -> bus_creator/15  "TesterPhysicalReqTCM"

== system test_mdl1/VehicleCAN/VDM ==
  Suspension_Data : Subsystem
  TesterPhysicalResVDM : Subsystem
  VeyDynamics_Data : Subsystem
  bus_creator : BusCreator  Inputs=3
  out_port : Outport
  wires:
  bus_creator/1 -> out_port/1  "test_mdl1"
  Suspension_Data/1(out_port) -> bus_creator/1  "Suspension_Data"
  TesterPhysicalResVDM/1(out_port) -> bus_creator/2  "TesterPhysicalResVDM"
  VeyDynamics_Data/1(out_port) -> bus_creator/3  "VeyDynamics_Data"

== system test_mdl1/VehicleCAN/ABS_ESC/ABS_AutoSar_NetworkMgt ==
  ABS_AutoSarNMNodeId : Constant  Value=0
  ABS_AutoSarNMReserved{1..4} (4 alike) : Constant  Value=0
  ABS_GWNMProxy : Constant  Value=0
  ABS_GWOnBoardTester : Constant  Value=0
  Constant : Constant
  bus_creator : BusCreator  Inputs=8
  out_port : Outport
  wires:
  bus_creator/1 -> out_port/1  "test_mdl1"
  ABS_AutoSarNMNodeId/1 -> bus_creator/2  "ABS_AutoSarNMNodeId"
  ABS_AutoSarNMReserved1/1 -> bus_creator/3  "ABS_AutoSarNMReserved1"
  ABS_AutoSarNMReserved2/1 -> bus_creator/4  "ABS_AutoSarNMReserved2"
  ABS_AutoSarNMReserved3/1 -> bus_creator/5  "ABS_AutoSarNMReserved3"
  ABS_AutoSarNMReserved4/1 -> bus_creator/6  "ABS_AutoSarNMReserved4"
  ABS_GWNMProxy/1 -> bus_creator/7  "ABS_GWNMProxy"
  ABS_GWOnBoardTester/1 -> bus_creator/8  "ABS_GWOnBoardTester"
  Constant/1 -> bus_creator/1  "ABS_AutoSarNMControl"

== system test_mdl1/VehicleCAN/ABS_ESC/ABS_BrkBst_Data ==
  BrkBstrVac_P_Actl : Constant  Value=0
  BrkHold_D_Stat : Constant  Value=0
  BrkTotTqRqDrv_No_Cnt : Constant  Value=0
  BrkTotTqRqDrv_No_Cs : Constant  Value=0
  BrkTot_Tq_RqDrv : Constant  Value=0
  HsaStat_D_Dsply : Constant  Value=0
  HsaTrnAout_Tq_Rq : Constant  Value=0
  YawStabilityIndex : Constant  Value=0
  bus_creator : BusCreator  Inputs=8
  out_port : Outport
  wires:
  bus_creator/1 -> out_port/1  "test_mdl1"
  BrkBstrVac_P_Actl/1 -> bus_creator/1  "BrkBstrVac_P_Actl"
  BrkHold_D_Stat/1 -> bus_creator/2  "BrkHold_D_Stat"
  BrkTotTqRqDrv_No_Cnt/1 -> bus_creator/3  "BrkTotTqRqDrv_No_Cnt"
  BrkTotTqRqDrv_No_Cs/1 -> bus_creator/4  "BrkTotTqRqDrv_No_Cs"
  BrkTot_Tq_RqDrv/1 -> bus_creator/5  "BrkTot_Tq_RqDrv"
  HsaStat_D_Dsply/1 -> bus_creator/6  "HsaStat_D_Dsply"
  HsaTrnAout_Tq_Rq/1 -> bus_creator/7  "HsaTrnAout_Tq_Rq"
  YawStabilityIndex/1 -> bus_creator/8  "YawStabilityIndex"

== system test_mdl1/VehicleCAN/ABS_ESC/ABS_Rapid_Data_Response_1 ==
  UUDTABSResponse1 : Constant  Value=0
  bus_creator : BusCreator  Inputs=1
  out_port : Outport
  wires:
  bus_creator/1 -> out_port/1  "test_mdl1"
  UUDTABSResponse1/1 -> bus_creator/1  "UUDTABSResponse1"
